simulink model "finalvers"  (R2023a)
settings: Solver=VariableStepAuto  StartTime=0.0  StopTime=10.0  FixedStep=0.0001  RelTol=1e-3
values from neighbouring files (symbols this model uses):
  ampl = 0.07    [stage1.m]
  beq = (((a/b)*cos(alpha))^2) * bd    [stage1.m]
  endt = 1.5    [stage1.m]
  keq = (((a/b)*cos(alpha))^2) * ks    [stage1.m]
  kT = 270*10^3    (= 270000)    [stage1.m]
  ms = 0.25*mv    (= 400)    [stage1.m]
  mu = 50    [stage1.m]
  startt = 0.5    [stage1.m]
  wavelength = 6    [stage1.m]
settings Model: Creator=Aditya  LastModifiedBy=u5529041

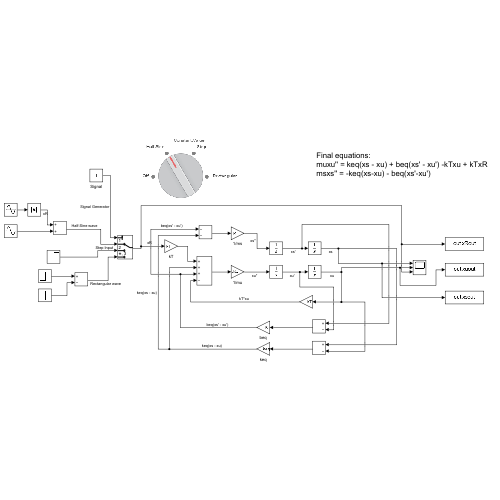
[thumbnail: Simulink's stored preview of the top-level diagram]
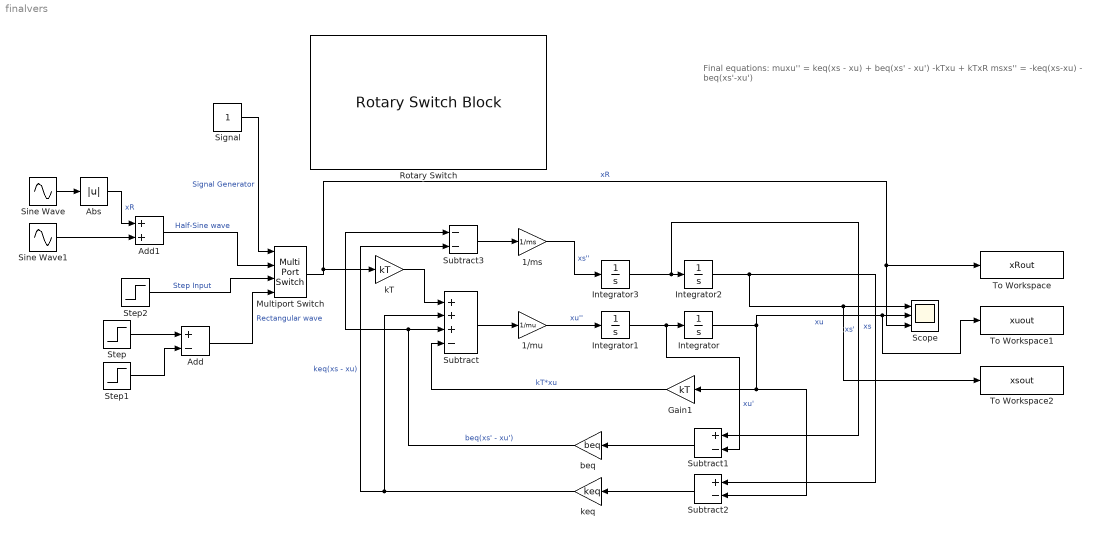
== system finalvers ==
  note: Final equations:
      | muxu'' = keq(xs - xu) + beq(xs' - xu') -kTxu + kTxR
      | msxs'' = -keq(xs-xu) - beq(xs'-xu')
  1/ms : Gain  Gain=1/ms
  1/mu : Gain  Gain=1/mu
  Abs : Abs  SaturateOnIntegerOverflow=off
  Add : Sum  Inputs=+-
  Add1 : Sum
  Gain1 : Gain  Gain=kT
  Integrator{,1..3} (4 alike) : Integrator
  Multiport Switch : MultiPortSwitch  SaturateOnIntegerOverflow=off  InputSameDT=off
  Rotary Switch : RotarySwitchBlock
      settings: Values={{'Off', 'Half-Sine', 'Step', 'Rectangular'}, [0 1 2 3]}
  Scope : Scope  NumInputPorts=3
  Signal : Constant
  Sine Wave : Sin  Amplitude=ampl  Frequency=2*pi/wavelength  SampleTime=0
  Sine Wave1 : Sin  Amplitude=ampl  Frequency=2*pi/wavelength  SampleTime=0
  Step : Step  Time=startt  After=0.12  SampleTime=0
  Step1 : Step  Time=endt  After=0.12  SampleTime=0
  Step2 : Step  SampleTime=0
  Subtract : Sum  Inputs=+++-
  Subtract1 : Sum  Inputs=+-
  Subtract2 : Sum  Inputs=+-
  Subtract3 : Sum  Inputs=--
  To Workspace : ToWorkspace  VariableName=xRout  SaveFormat=Timeseries  SampleTime=-1
  To Workspace1 : ToWorkspace  VariableName=xuout  SaveFormat=Timeseries  SampleTime=-1
  To Workspace2 : ToWorkspace  VariableName=xsout  SaveFormat=Timeseries  SampleTime=-1
  beq : Gain  Gain=beq
  kT : Gain  Gain=kT
  keq : Gain  Gain=keq
  wires:
  Multiport Switch/1 -> Scope/3, To Workspace/1, kT/1  "xR"
  Integrator/1 -> Subtract2/2, Gain1/1, To Workspace1/1, Scope/2  "xu"
  Integrator1/1 -> Subtract1/2, Integrator/1  "xu'"
  kT/1 -> Subtract/1
  Gain1/1 -> Subtract/4  "kT*xu"
  Integrator2/1 -> Subtract2/1, To Workspace2/1, Scope/1  "xs"
  Integrator3/1 -> Subtract1/1, Integrator2/1  "xs'"
  Subtract1/1 -> beq/1
  beq/1 -> Subtract3/1, Subtract/3  "beq(xs' - xu')"
  Subtract2/1 -> keq/1
  keq/1 -> Subtract/2, Subtract3/2  "keq(xs - xu)"
  Subtract/1 -> 1/mu/1
  1/mu/1 -> Integrator1/1  "xu''"
  Subtract3/1 -> 1/ms/1
  1/ms/1 -> Integrator3/1  "xs''"
  Step/1 -> Add/1
  Step1/1 -> Add/2
  Sine Wave/1 -> Abs/1
  Abs/1 -> Add1/1  "xR"
  Sine Wave1/1 -> Add1/2
  Add1/1 -> Multiport Switch/2  "Half-Sine wave"
  Add/1 -> Multiport Switch/4  "Rectangular wave"
  Step2/1 -> Multiport Switch/3  "Step Input"
  Signal/1 -> Multiport Switch/1  "Signal Generator"
